simulink model "FieldControl_PID"  (R2021a)
settings: Solver=ode45  StartTime=0.0  StopTime=3  FixedStep=1e-5  MaxStep=1e-6  RelTol=1e-3
model workspace (MAT data in the model file):
  KI_s = 1
  KP_s = 1
undefined symbols (not defined in the file): DiscIntNeverNeededParam, Fsw, sigbuilder_block
libraries: simulink x2, spspowerguiLib x2
(part 1 of 2)
settings Model: SimulationMode=accelerator  OrderedModelArguments=off  Creator=AHMED  LastModifiedBy=AHMED
settings SolverCC: ZeroCrossAlgorithm=Adaptive
settings DebuggingCC: MaskedZcDiagnostic=none  IgnoredZcDiagnostic=none

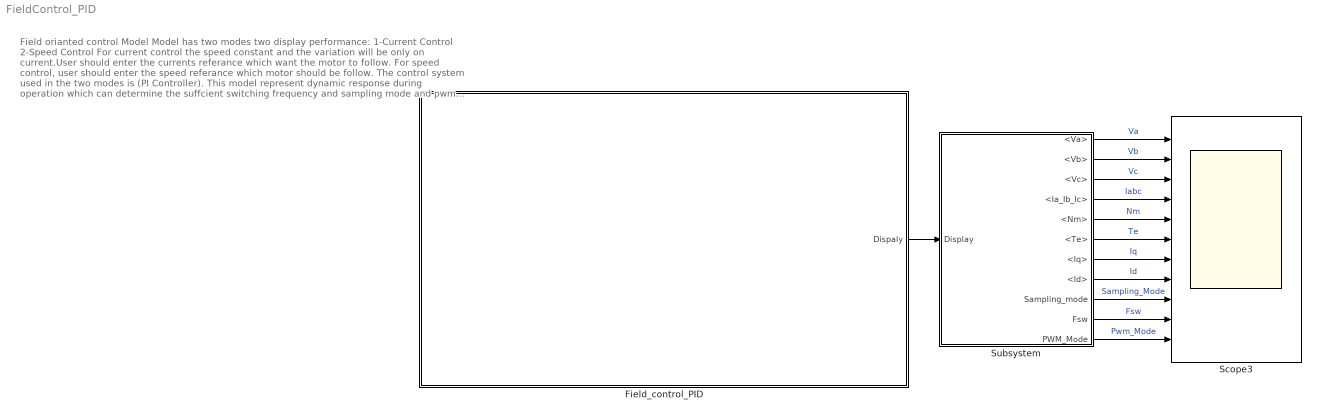
== system FieldControl_PID ==
  note: Field orianted control Model
      | Model has two modes two display performance:
      | 1-Current Control
      | 2-Speed Control
      | For current control the speed constant and the variation will be only on current.User should enter the currents referance which want the motor to follow.
      |
      | For speed control, user should enter the speed referance which motor should be follow.
      |
      | The control system used in the two modes is (PI Controller).
      |
      | This model represent dynamic response during operation which can determine the suffcient switching frequency and sampling mode and pwm generation technique.
      |
      | The dynamical behaviour according to the best performance and lower losses could be achieved.
      |
      | PWM generating techniques
      | 1-Space Vector Modulation(SVM)
      | 2-General Discontinous PWM (GDPWM)
      |
      | Sampling Modes
      | 1-Symmetrical Sampling Mode
      | 2-Asymmetrical Sampling Mode
      |
      | Selected switching frequency according fundmental frequency measured from the operating speed and it has low and high limits.
  Field_control_PID : Subsystem  Variant=on  mask{Mode=Speed_Control, Vdc=400, PWM_Mode=Auto, Sw2fund_Ration=50, Lower_Limit=4e3, Higher_Limit=10e3, Typee=Equations, TL=0.75, Nm_CC=1200}
      mask prompts: Mode "Control_System"; Vdc "DC voltage"; PWM_Mode "PWM_Generation_Mode"; Sw2fund_Ration "Switching to fund_ freq Ratio"; Lower_Limit "Lower Limit"; Typee "MTPA_System"; TL "Load Torque"; Nm_CC "Constant_Speed_RPM"
      mask TypeOptions Mode: Current_Control | Speed_Control
      mask TypeOptions PWM_Mode: SVM | DPWM | Auto
      mask TypeOptions Typee: Equations | Tables
      mask DialogControl DescGroupVar Prompt: FOC_PMSM_parameters
      mask DialogControl DescTextVar Prompt: Field orianted control with two modes of operation (current, speed)control. Each one has parametrs must be input before run
      mask DialogControl ParameterGroupVar Prompt: Control Type & Motor parameters
      mask DialogControl ParameterGroupVar2 Prompt: Frequency and sampling
      mask DialogControl ParameterGroupVar3 Prompt: Speed control parameters
      mask DialogControl ParameterGroupVar4 Prompt: Current control parameters
      mask Display: image('$imagefile'); % Use "Edit Image" on toolstrip to change.
  Scope3 : Scope  NumInputPorts=11
  Subsystem : Subsystem
      mask Display: image('$imagefile'); % Use "Edit Image" on toolstrip to change.
  wires:
  Field_control_PID/1(Dispaly) -> Subsystem/1(Display)
  Subsystem/1(<Va>) -> Scope3/1  "Va"
  Subsystem/2(<Vb>) -> Scope3/2  "Vb"
  Subsystem/3(<Vc>) -> Scope3/3  "Vc"
  Subsystem/4(<Ia_Ib_Ic>) -> Scope3/4  "Iabc"
  Subsystem/5(<Nm>) -> Scope3/5  "Nm"
  Subsystem/6(<Te>) -> Scope3/6  "Te"
  Subsystem/7(<Iq>) -> Scope3/7  "Iq"
  Subsystem/8(<Id>) -> Scope3/8  "Id"
  Subsystem/9(Sampling_mode) -> Scope3/9  "Sampling_Mode"
  Subsystem/10(Fsw) -> Scope3/10  "Fsw"
  Subsystem/11(PWM_Mode) -> Scope3/11  "Pwm_Mode"

== system FieldControl_PID/Field_control_PID ==
  Current_control : Subsystem  VariantControl=Mode==1
  Speed_control : Subsystem  VariantControl=Mode==2
  Dispaly : Outport

== system FieldControl_PID/Subsystem ==
  Display : Inport
  Bus Selector : BusSelector  OutputSignals=Va,Vb,Vc,Ia_Ib_Ic,Nm,Te,Iq,Id,sampling_Mode,Fswitching,PWM_Gen_Mode
  Constant : Constant  Value=2
  Constant1 : Constant
  Constant2 : Constant  Value=4e3
  Constant3 : Constant  Value=10e3
  Constant4 : Constant  Value=0
  Constant5 : Constant
  Mux : Mux  Inputs=3
  Mux1 : Mux  Inputs=3
  Mux2 : Mux  Inputs=3
  <Va> : Outport
  <Vb> : Outport  Port=2
  <Vc> : Outport  Port=3
  <Ia_Ib_Ic> : Outport  Port=4
  <Nm> : Outport  Port=5
  <Te> : Outport  Port=6
  <Iq> : Outport  Port=7
  <Id> : Outport  Port=8
  Sampling_mode : Outport  Port=9
  Fsw : Outport  Port=10
  PWM_Mode : Outport  Port=11
  wires:
  Bus Selector/10 -> Mux1/1  "<Fswitching>"
  Constant5/1 -> Mux2/3  "GDPWM"
  Constant2/1 -> Mux1/2  "Lower_Limit"
  Constant/1 -> Mux/2  "Symmetrical"
  Bus Selector/11 -> Mux2/1  "<PWM_Gen_Mode>"
  Constant1/1 -> Mux/3  "Asymmetrical"
  Bus Selector/6 -> <Te>/1  "<Te>"
  Constant3/1 -> Mux1/3  "Upper_Limit"
  Display/1 -> Bus Selector/1
  Bus Selector/9 -> Mux/1  "<sampling_Mode>"
  Constant4/1 -> Mux2/2  "SVM"
  Bus Selector/8 -> <Id>/1  "<Id>"
  Bus Selector/5 -> <Nm>/1  "<Nm>"
  Bus Selector/1 -> <Va>/1  "<Va>"
  Mux/1 -> Sampling_mode/1  "Sampling_mode"
  Bus Selector/3 -> <Vc>/1  "<Vc>"
  Bus Selector/4 -> <Ia_Ib_Ic>/1  "<Ia_Ib_Ic>"
  Bus Selector/2 -> <Vb>/1  "<Vb>"
  Bus Selector/7 -> <Iq>/1  "<Iq>"
  Mux1/1 -> Fsw/1
  Mux2/1 -> PWM_Mode/1  "PWM_Mode"

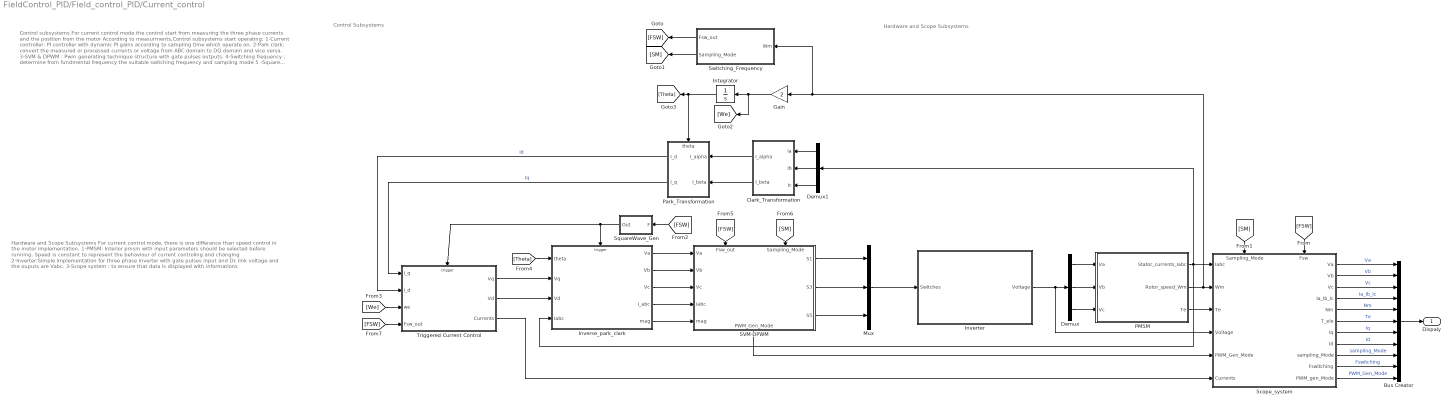
== system FieldControl_PID/Field_control_PID/Current_control ==
  note: Control subsystems
      | For current control mode the control start from measuring the three phase currents and the position from the motor
      | According to measurments,Control subsystems start operating:
      | 1-Current controller: PI controller with dynamic PI gains according to sampling time which operate on.
      |
      | 2-Park clark: convert the measured or processed currents or voltage
      | from ABC domain to DQ domain and vice versa.
      |
      | 3-SVM & DPWM : Pwm generating technique structure with gate pulses outputs.
      |
      | 4-Switching frequency : determine from fundmental frequency the suitable switching frequency and sampling mode
      |
      | 5 -Square Wave generator: with frequency input
  note: Hardware and Scope Subsystems
  note: Control Subsystems
  note: Hardware and Scope Subsystems
      | For current control mode, there is one differance than speed control in the motor implementation.
      | 1-PMSM: Interior pmsm with input parameters should be selected before running.
      | Speed is constant to represent the behaviour of current controling and changing
      |
      | 2-Inverter:Simple implementation for three phase inverter with gate pulses input and Dc link voltage and the ouputs are Vabc.
      |
      | 3-Scope system : to ensure that data is displayed with informations
  Bus Creator : BusCreator  Inputs=11
  Clark_Transformation : Subsystem
  Demux : Demux  Outputs=3
  Demux1 : Demux  Outputs=3
  Gain : Gain  Gain=2
  Integrator : Integrator
  Inverse_park_clark : Subsystem
  "Inverter " : Subsystem
      mask Display: image('E:\matlab_modules\FOC_PMSM\Final_1_FOC_PMSM\Images\WhatsApp Image 2024-10-21 at 22.54.49_e8a4c1c9.jpg'); % Use "Edit Image" on toolstrip to change.
  Mux : Mux  Inputs=3
  PMSM : Subsystem  mask{Ld=0.0057, Lq=0.0125, lamda_pm=0.123, R=1.2, P=4, J=0.0001, b=0}
      mask Display: image('$imagefile'); % Use "Edit Image" on toolstrip to change.
  Park_Transformation : Subsystem
      settings: PortSchema="{\"entries\":[{\"content\":{\"sides\":[{\"content\":{\"connectorIds\":[\"In1\",\"In2\"]},\"type\":\"ConnectorPlacement.EquallySpacedRectSide\",\"uuid\":\"a5303260-9056-4ba9-bf21-9d9e68c76aad\"},{\"content\":{\"connectorIds\":[\"Out1\",\"Out2\"],\"side\":\"RIGHT\"},\"type\":\"ConnectorPlacement.EquallySpacedRectSide\",\"uuid\":\"bf8eba39-f781-4672-b99d-9d1cb4b6396f\"},{\"content\":{\"connectorIds\":[\"In3\"],\"side\":\"TOP\"},\"type\":\"ConnectorPlacement.EquallySpacedRectSide\",\"uuid\":\"4985423e-053d-4914-82fe-b9dd9f427f0d\"},{\"content\":{\"connectorIds\":[],\"side\":\"BOTTOM\"},\"type\":\"ConnectorPlacement.EquallySpacedRectSide\",\"uuid\":\"0752c2be-c5bb-44b3-a6b0-4f5b66c2ccb1\"}]},\"type\":\"ConnectorPlacement.EquallySpacedConnector\",\"uuid\":\"0aeb7acd-9c9e-4bf3-9d65-4f157eb3bd0a\"}],\"packageUris\":[\"http://schema.mathworks.com/mf0/Connector/R2020b\"],\"version\":\"1.0\"}"
  SVM-DPWM : Subsystem
      settings: PortSchema="{\"entries\":[{\"content\":{\"sides\":[{\"content\":{\"connectorIds\":[\"In1\",\"In2\",\"In3\",\"In4\",\"In5\"]},\"type\":\"ConnectorPlacement.EquallySpacedRectSide\",\"uuid\":\"46ad86bc-2290-42eb-9805-a724d3d45e27\"},{\"content\":{\"connectorIds\":[\"Out1\",\"Out2\",\"Out3\"],\"side\":\"RIGHT\"},\"type\":\"ConnectorPlacement.EquallySpacedRectSide\",\"uuid\":\"f1ee6116-553b-4cc4-988e-efe9f7b6e0cc\"},{\"content\":{\"connectorIds\":[\"In6\",\"In7\"],\"side\":\"TOP\"},\"type\":\"ConnectorPlacement.EquallySpacedRectSide\",\"uuid\":\"0619aa55-dbb7-4591-ac57-1e3d225085e5\"},{\"content\":{\"connectorIds\":[\"Out4\"],\"side\":\"BOTTOM\"},\"type\":\"ConnectorPlacement.EquallySpacedRectSide\",\"uuid\":\"7325c7f4-f74c-41be-974a-a0e5e3a4c9b0\"}]},\"type\":\"ConnectorPlacement.EquallySpacedConnector\",\"uuid\":\"4aef647a-1044-4613-b672-2a7f7848e9d8\"}],\"packageUris\":[\"http://schema.mathworks.com/mf0/Connector/R2020b\"],\"version\":\"1.0\"}"
      mask Display: image('E:\matlab_modules\FOC_PMSM\Final_1_FOC_PMSM\Images\photo_2024-12-25_16-03-35.jpg'); % Use "Edit Image" on toolstrip to change.
  Scope_system : Subsystem
      settings: PortSchema="{\"entries\":[{\"content\":{\"sides\":[{\"content\":{\"connectorIds\":[\"In1\",\"In2\",\"In3\",\"In4\",\"In5\",\"In6\"]},\"type\":\"ConnectorPlacement.EquallySpacedRectSide\",\"uuid\":\"f5ff00d6-72d0-455a-b8b4-a2b5e0f936c9\"},{\"content\":{\"connectorIds\":[\"Out1\",\"Out2\",\"Out3\",\"Out4\",\"Out5\",\"Out6\",\"Out7\",\"Out8\",\"Out9\",\"Out10\",\"Out11\"],\"side\":\"RIGHT\"},\"type\":\"ConnectorPlacement.EquallySpacedRectSide\",\"uuid\":\"90221681-7e43-47d8-9ea8-4435eb27af9a\"},{\"content\":{\"connectorIds\":[\"In7\",\"In8\"],\"side\":\"TOP\"},\"type\":\"ConnectorPlacement.EquallySpacedRectSide\",\"uuid\":\"62fb04f8-341d-442a-bb15-2a5c062453bf\"}]},\"type\":\"ConnectorPlacement.EquallySpacedConnector\",\"uuid\":\"244d1d3d-d937-49d8-9876-c8777bd7e7cc\"}],\"packageUris\":[\"http://schema.mathworks.com/mf0/Connector/R2020b\"],\"version\":\"1.0\"}"
      mask Display: image('$imagefile'); % Use "Edit Image" on toolstrip to change.
  SquareWave_Gen : Subsystem
  Switching_Frequency : Subsystem
  Triggered Current Control : Subsystem  TreatAsAtomicUnit=on
  Dispaly : Outport
  wires:
  Demux1/3 -> Clark_Transformation/3(Ic)
  Demux1/1 -> Clark_Transformation/1(Ia)
  Scope_system/8("Id ") -> Bus Creator/8  "Id"
  Scope_system/7(Iq) -> Bus Creator/7  "Iq"
  Clark_Transformation/1(I_alpha) -> Park_Transformation/1(I_alpha)
  Scope_system/3(Vc) -> Bus Creator/3  "Vc"
  Clark_Transformation/2(I_beta) -> Park_Transformation/2(I_beta)
  Demux1/2 -> Clark_Transformation/2(Ib)
  Bus Creator/1 -> Dispaly/1
  Scope_system/1(Va) -> Bus Creator/1  "Va"
  Scope_system/4(Ia_Ib_Ic) -> Bus Creator/4  "Ia_Ib_Ic"
  Scope_system/2(Vb) -> Bus Creator/2  "Vb"
  Scope_system/5(Nm) -> Bus Creator/5  "Nm"
  Scope_system/6(T_ele) -> Bus Creator/6  "Te"
  Scope_system/9(sampling_Mode) -> Bus Creator/9  "sampling_Mode"
  Scope_system/10(Fswitching) -> Bus Creator/10  "Fswitching"
  Scope_system/11(PWM_gen_Mode) -> Bus Creator/11  "PWM_Gen_Mode"
  SVM-DPWM/1(S1) -> Mux/1
  SVM-DPWM/2(S3) -> Mux/2
  SVM-DPWM/3(S5) -> Mux/3
  Mux/1 -> "Inverter "/1("Switches ")
  "Inverter "/1("Voltage ") -> Scope_system/4("Voltage "), Demux/1
  Demux/1 -> PMSM/1(Va)
  Demux/2 -> PMSM/2(Vb)
  Demux/3 -> PMSM/3(Vc)
  Inverse_park_clark/1(Va) -> SVM-DPWM/1(Va)
  Inverse_park_clark/2(Vb) -> SVM-DPWM/2(Vb)
  Inverse_park_clark/3(Vc) -> SVM-DPWM/3(Vc)
  Inverse_park_clark/4(I_abc) -> SVM-DPWM/4(Iabc)
  Inverse_park_clark/5(mag) -> SVM-DPWM/5(mag)
  Triggered Current Control/1(Vq) -> Inverse_park_clark/2(Vq)
  Triggered Current Control/2(Vd) -> Inverse_park_clark/3(Vd)
  Gain/1 -> [We], Integrator/1
  Integrator/1 -> [Theta], Park_Transformation/3(theta)
  Switching_Frequency/1(Fsw_out) -> [FSW]
  Switching_Frequency/2(Sampling_Mode) -> [SM]
  [Theta] -> Inverse_park_clark/1(theta)
  Park_Transformation/2(I_q) -> Triggered Current Control/1(I_q)  "Iq"
  Park_Transformation/1(I_d) -> Triggered Current Control/2(I_d)  "Id"
  [FSW] -> SquareWave_Gen/1(F)
  SquareWave_Gen/1(Out) -> Inverse_park_clark/Trigger, Triggered Current Control/Trigger
  [We] -> Triggered Current Control/3(we)
  [SM] -> Scope_system/7(Sampling_Mode)
  [FSW] -> Scope_system/8(Fsw)
  [SM] -> SVM-DPWM/7(Sampling_Mode)
  [FSW] -> SVM-DPWM/6(Fsw_out)
  [FSW] -> Triggered Current Control/4(Fsw_out)
  PMSM/1(Stator_currents_Iabc) -> Inverse_park_clark/4(Iabc), Scope_system/1(Iabc), Demux1/1
  PMSM/2(Rotor_speed_Wm) -> Switching_Frequency/1(Wm), Gain/1, Scope_system/2(Wm)
  PMSM/3(Te) -> Scope_system/3(Te)
  Triggered Current Control/3(Currents) -> Scope_system/6(Currents)
  SVM-DPWM/4(PWM_Gen_Mode) -> Scope_system/5(PWM_Gen_Mode)

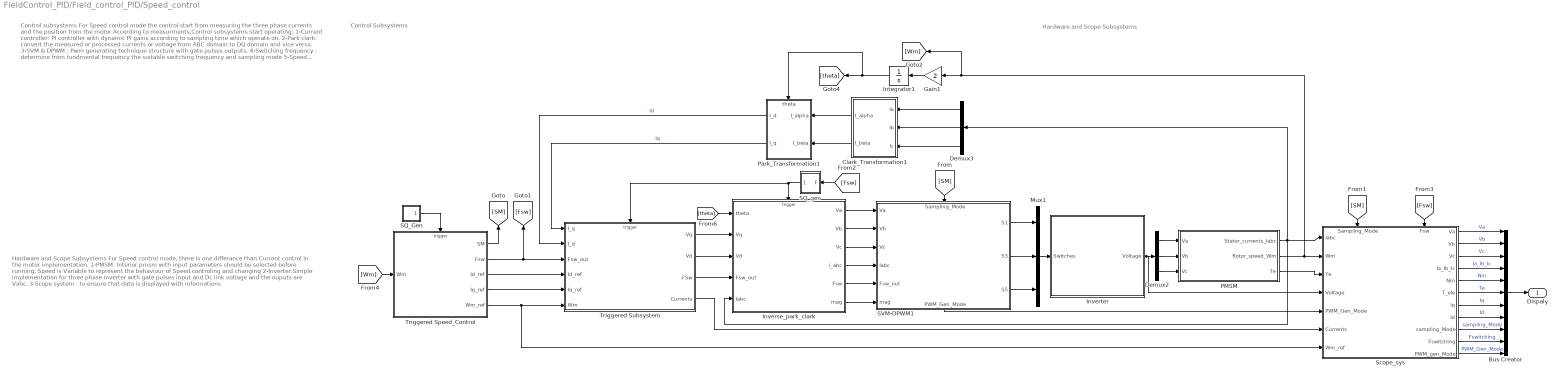
== system FieldControl_PID/Field_control_PID/Speed_control ==
  note: Hardware and Scope Subsystems
  note: Control Subsystems
  note: Control subsystems
      | For Speed control mode the control start from measuring the three phase currents and the position from the motor
      | According to measurments,Control subsystems start operating:
      | 1-Current controller: PI controller with dynamic PI gains according to sampling time which operate on.
      |
      | 2-Park clark: convert the measured or processed currents or voltage
      | from ABC domain to DQ domain and vice versa.
      |
      | 3-SVM & DPWM : Pwm generating technique structure with gate pulses outputs.
      |
      | 4-Switching frequency : determine from fundmental frequency the suitable switching frequency and sampling mode
      |
      | 5-Speed Controller: PI controller with constant PI gains.
      |
      | 6-Square Wave generator: with frequency input
  note: Hardware and Scope Subsystems
      | For Speed control mode, there is one differance than Current control in the motor implementation.
      | 1-PMSM: Interior pmsm with input parameters should be selected before running.
      | Speed is Variable to represent the behaviour of Speed controling and changing
      |
      | 2-Inverter:Simple implementation for three phase inverter with gate pulses input and Dc link voltage and the ouputs are Vabc.
      |
      | 3-Scope system : to ensure that data is displayed with informations
  Bus Creator : BusCreator  Inputs=11
  Clark_Transformation1 : Subsystem
  Demux2 : Demux  Outputs=3
  Demux3 : Demux  Outputs=3
  Gain1 : Gain  Gain=2
  Integrator1 : Integrator
  Inverse_park_clark : Subsystem
  "Inverter " : Subsystem
      mask Display: image('$imagefile'); % Use "Edit Image" on toolstrip to change.
  Mux1 : Mux  Inputs=3
  PMSM : Subsystem  mask{Ld=0.0057, Lq=0.0125, lamda_pm=0.123, R=1.2, P=4, J=0.0001, b=0}
      mask Display: image('$imagefile'); % Use "Edit Image" on toolstrip to change.
  Park_Transformation1 : Subsystem
      settings: PortSchema="{\"entries\":[{\"content\":{\"sides\":[{\"content\":{\"connectorIds\":[\"In1\",\"In2\"]},\"type\":\"ConnectorPlacement.EquallySpacedRectSide\",\"uuid\":\"a5303260-9056-4ba9-bf21-9d9e68c76aad\"},{\"content\":{\"connectorIds\":[\"Out1\",\"Out2\"],\"side\":\"RIGHT\"},\"type\":\"ConnectorPlacement.EquallySpacedRectSide\",\"uuid\":\"bf8eba39-f781-4672-b99d-9d1cb4b6396f\"},{\"content\":{\"connectorIds\":[\"In3\"],\"side\":\"TOP\"},\"type\":\"ConnectorPlacement.EquallySpacedRectSide\",\"uuid\":\"4985423e-053d-4914-82fe-b9dd9f427f0d\"},{\"content\":{\"connectorIds\":[],\"side\":\"BOTTOM\"},\"type\":\"ConnectorPlacement.EquallySpacedRectSide\",\"uuid\":\"0752c2be-c5bb-44b3-a6b0-4f5b66c2ccb1\"}]},\"type\":\"ConnectorPlacement.EquallySpacedConnector\",\"uuid\":\"0aeb7acd-9c9e-4bf3-9d65-4f157eb3bd0a\"}],\"packageUris\":[\"http://schema.mathworks.com/mf0/Connector/R2020b\"],\"version\":\"1.0\"}"
  SQ_Gen : Subsystem
  SQ_gen : Subsystem
  SVM-DPWM1 : Subsystem
      settings: PortSchema="{\"entries\":[{\"content\":{\"sides\":[{\"content\":{\"connectorIds\":[\"In1\",\"In2\",\"In3\",\"In4\",\"In5\",\"In6\"]},\"type\":\"ConnectorPlacement.EquallySpacedRectSide\",\"uuid\":\"46ad86bc-2290-42eb-9805-a724d3d45e27\"},{\"content\":{\"connectorIds\":[\"Out1\",\"Out2\",\"Out3\"],\"side\":\"RIGHT\"},\"type\":\"ConnectorPlacement.EquallySpacedRectSide\",\"uuid\":\"f1ee6116-553b-4cc4-988e-efe9f7b6e0cc\"},{\"content\":{\"connectorIds\":[\"In7\"],\"side\":\"TOP\"},\"type\":\"ConnectorPlacement.EquallySpacedRectSide\",\"uuid\":\"0619aa55-dbb7-4591-ac57-1e3d225085e5\"},{\"content\":{\"connectorIds\":[\"Out4\"],\"side\":\"BOTTOM\"},\"type\":\"ConnectorPlacement.EquallySpacedRectSide\",\"uuid\":\"7325c7f4-f74c-41be-974a-a0e5e3a4c9b0\"}]},\"type\":\"ConnectorPlacement.EquallySpacedConnector\",\"uuid\":\"4aef647a-1044-4613-b672-2a7f7848e9d8\"}],\"packageUris\":[\"http://schema.mathworks.com/mf0/Connector/R2020b\"],\"version\":\"1.0\"}"
      mask Display: image('$imagefile'); % Use "Edit Image" on toolstrip to change.
  Scope_sys : Subsystem
      settings: PortSchema="{\"entries\":[{\"content\":{\"sides\":[{\"content\":{\"connectorIds\":[\"In1\",\"In2\",\"In3\",\"In4\",\"In5\",\"In6\",\"In7\"]},\"type\":\"ConnectorPlacement.EquallySpacedRectSide\",\"uuid\":\"f5ff00d6-72d0-455a-b8b4-a2b5e0f936c9\"},{\"content\":{\"connectorIds\":[\"Out1\",\"Out2\",\"Out3\",\"Out4\",\"Out5\",\"Out6\",\"Out7\",\"Out8\",\"Out9\",\"Out10\",\"Out11\"],\"side\":\"RIGHT\"},\"type\":\"ConnectorPlacement.EquallySpacedRectSide\",\"uuid\":\"90221681-7e43-47d8-9ea8-4435eb27af9a\"},{\"content\":{\"connectorIds\":[\"In8\",\"In9\"],\"side\":\"TOP\"},\"type\":\"ConnectorPlacement.EquallySpacedRectSide\",\"uuid\":\"62fb04f8-341d-442a-bb15-2a5c062453bf\"}]},\"type\":\"ConnectorPlacement.EquallySpacedConnector\",\"uuid\":\"244d1d3d-d937-49d8-9876-c8777bd7e7cc\"}],\"packageUris\":[\"http://schema.mathworks.com/mf0/Connector/R2020b\"],\"version\":\"1.0\"}"
      mask Display: image('$imagefile'); % Use "Edit Image" on toolstrip to change.
  Triggered Speed_Control : Subsystem  TreatAsAtomicUnit=on
  Triggered Subsystem : Subsystem  TreatAsAtomicUnit=on
  Dispaly : Outport
  wires:
  "Inverter "/1("Voltage ") -> Scope_sys/4("Voltage "), Demux2/1
  Demux3/1 -> Clark_Transformation1/1(Ia)
  Scope_sys/8("Id ") -> Bus Creator/8  "Id"
  Scope_sys/7(Iq) -> Bus Creator/7  "Iq"
  Demux3/3 -> Clark_Transformation1/3(Ic)
  Scope_sys/6(T_ele) -> Bus Creator/6  "Te"
  Scope_sys/3(Vc) -> Bus Creator/3  "Vc"
  Scope_sys/5(Nm) -> Bus Creator/5  "Nm"
  Scope_sys/2(Vb) -> Bus Creator/2  "Vb"
  Scope_sys/10(Fswitching) -> Bus Creator/10  "Fswitching"
  Scope_sys/1(Va) -> Bus Creator/1  "Va"
  Mux1/1 -> "Inverter "/1("Switches ")
  Demux3/2 -> Clark_Transformation1/2(Ib)
  Clark_Transformation1/1(I_alpha) -> Park_Transformation1/1(I_alpha)
  Scope_sys/9(sampling_Mode) -> Bus Creator/9  "sampling_Mode"
  Clark_Transformation1/2(I_beta) -> Park_Transformation1/2(I_beta)
  Bus Creator/1 -> Dispaly/1
  Scope_sys/4(Ia_Ib_Ic) -> Bus Creator/4  "Ia_Ib_Ic"
  [SM] -> SVM-DPWM1/7(Sampling_Mode)
  [SM] -> Scope_sys/8(Sampling_Mode)
  SQ_gen/1(Cs) -> Triggered Subsystem/Trigger, Inverse_park_clark/Trigger
  [Fsw] -> SQ_gen/1(F)
  [Fsw] -> Scope_sys/9(Fsw)
  [theta] -> Inverse_park_clark/1(theta)
  Scope_sys/11(PWM_gen_Mode) -> Bus Creator/11  "PWM_Gen_Mode"
  PMSM/1(Stator_currents_Iabc) -> Demux3/1, Scope_sys/1(Iabc), Inverse_park_clark/5(Iabc)
  PMSM/2(Rotor_speed_Wm) -> [Wm], Gain1/1, Scope_sys/2(Wm)
  PMSM/3(Te) -> Scope_sys/3(Te)
  Demux2/1 -> PMSM/1(Va)
  Demux2/2 -> PMSM/2(Vb)
  Demux2/3 -> PMSM/3(Vc)
  SVM-DPWM1/1(S1) -> Mux1/1
  SVM-DPWM1/2(S3) -> Mux1/2
  SVM-DPWM1/3(S5) -> Mux1/3
  Inverse_park_clark/1(Va) -> SVM-DPWM1/1(Va)
  Inverse_park_clark/2(Vb) -> SVM-DPWM1/2(Vb)
  Inverse_park_clark/3(Vc) -> SVM-DPWM1/3(Vc)
  Inverse_park_clark/4(i_abc) -> SVM-DPWM1/4(Iabc)
  Inverse_park_clark/5(Fsw) -> SVM-DPWM1/5(Fsw_out)
  Inverse_park_clark/6(mag) -> SVM-DPWM1/6(mag)
  Triggered Subsystem/1(Vq) -> Inverse_park_clark/2(Vq)
  Triggered Subsystem/2(Vd) -> Inverse_park_clark/3(Vd)
  Triggered Subsystem/3(FSw) -> Inverse_park_clark/4(Fsw_out)
  Integrator1/1 -> Park_Transformation1/3(theta), [theta]
  Gain1/1 -> Integrator1/1
  Triggered Subsystem/4(Currents) -> Scope_sys/6(Currents)
  SVM-DPWM1/4(PWM_Gen_Mode) -> Scope_sys/5(PWM_Gen_Mode)
  Triggered Speed_Control/2(Fsw) -> [Fsw], Triggered Subsystem/3(Fsw_out)
  Triggered Speed_Control/3(Id_ref) -> Triggered Subsystem/4(Id_ref)
  Triggered Speed_Control/4(Iq_ref) -> Triggered Subsystem/5(Iq_ref)
  Triggered Speed_Control/5(Wm_ref) -> Triggered Subsystem/6(Wm), Scope_sys/7(Wm_ref)
  Triggered Speed_Control/1(SM) -> [SM]
  [Wm] -> Triggered Speed_Control/1(Wm)
  Park_Transformation1/2(I_q) -> Triggered Subsystem/1(I_q)  "Iq"
  Park_Transformation1/1(I_d) -> Triggered Subsystem/2(I_d)  "Id"
  SQ_Gen/1(Cs) -> Triggered Speed_Control/Trigger

== system FieldControl_PID/Field_control_PID/Current_control/Clark_Transformation ==
  Ia : Inport
  Ib : Inport  Port=2
  Ic : Inport  Port=3
  Add : Sum  Inputs=+++
  Add1 : Sum
  Gain : Gain  Gain=-0.5
  Gain1 : Gain  Gain=-0.5
  Gain2 : Gain  Gain=2/3
  Gain3 : Gain  Gain=sqrt(3)/2
  Gain4 : Gain  Gain=-sqrt(3)/2
  Gain5 : Gain  Gain=2/3
  I_alpha : Outport
  I_beta : Outport  Port=2
  wires:
  Gain5/1 -> I_beta/1
  Add1/1 -> Gain5/1
  Gain3/1 -> Add1/1
  Gain4/1 -> Add1/2
  Gain2/1 -> I_alpha/1
  Add/1 -> Gain2/1
  Ia/1 -> Add/1
  Gain1/1 -> Add/3
  Gain/1 -> Add/2
  Ic/1 -> Gain1/1, Gain4/1
  Ib/1 -> Gain/1, Gain3/1

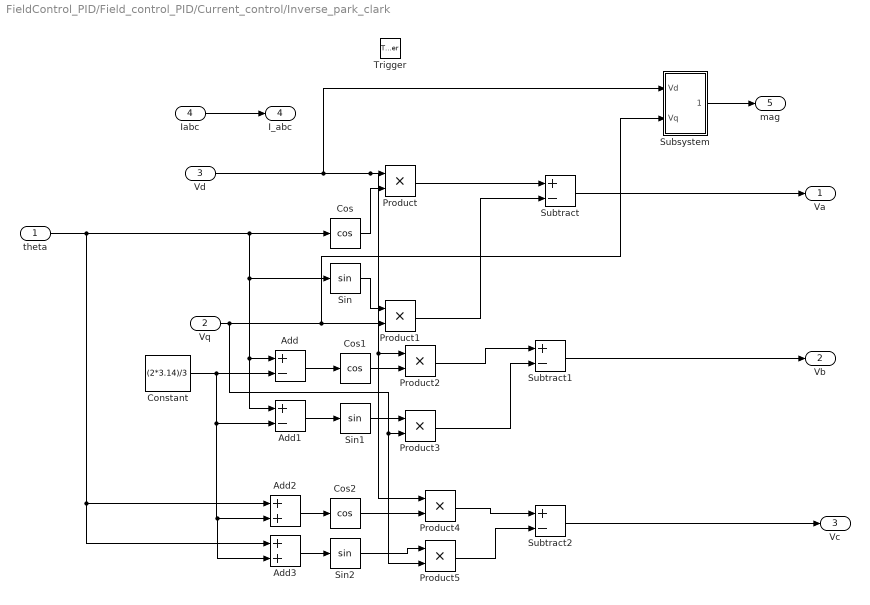
== system FieldControl_PID/Field_control_PID/Current_control/Inverse_park_clark ==
  theta : Inport
  Vq : Inport  Port=2
  Vd : Inport  Port=3
  Iabc : Inport  Port=4
  Trigger : TriggerPort  VariantControl=(inherit)
  Add : Sum  Inputs=+-
  Add1 : Sum  Inputs=+-
  Add2 : Sum
  Add3 : Sum
  Constant : Constant  Value=(2*3.14)/3
  Cos : Trigonometry  Operator=cos
  Cos1 : Trigonometry  Operator=cos
  Cos2 : Trigonometry  Operator=cos
  Product{,1..5} (6 alike) : Product
  Sin : Trigonometry
  Sin1 : Trigonometry
  Sin2 : Trigonometry
  Subsystem : Subsystem
  Subtract : Sum  Inputs=+-
  Subtract1 : Sum  Inputs=+-
  Subtract2 : Sum  Inputs=+-
  Va : Outport
  Vb : Outport  Port=2
  Vc : Outport  Port=3
  I_abc : Outport  Port=4
  mag : Outport  Port=5
  wires:
  Add3/1 -> Sin2/1
  Add2/1 -> Cos2/1
  Sin2/1 -> Product5/1
  Cos2/1 -> Product4/2
  Product5/1 -> Subtract2/2
  Product4/1 -> Subtract2/1
  Subtract2/1 -> Vc/1
  Constant/1 -> Add/2, Add1/2, Add2/2, Add3/2
  Subtract1/1 -> Vb/1
  Product3/1 -> Subtract1/2
  Product2/1 -> Subtract1/1
  Sin1/1 -> Product3/1
  Cos1/1 -> Product2/2
  Add1/1 -> Sin1/1
  Add/1 -> Cos1/1
  Product1/1 -> Subtract/2
  Sin/1 -> Product1/1
  Vq/1 -> Subsystem/2(Vq), Product1/2, Product3/2, Product5/2
  Product/1 -> Subtract/1
  Cos/1 -> Product/2
  Vd/1 -> Subsystem/1(Vd), Product/1, Product2/1, Product4/1
  theta/1 -> Sin/1, Add/1, Add1/1, Cos/1, Add2/1, Add3/1
  Subtract/1 -> Va/1
  Iabc/1 -> I_abc/1
  Subsystem/1(mag) -> mag/1

== system FieldControl_PID/Field_control_PID/Current_control/Inverter  ==
  "Switches " : Inport
  Fcn : Fcn  Expr=Vdc/3*(2*u(1)-u(2)-u(3))
  Fcn1 : Fcn  Expr=Vdc/3*(2*u(2)-u(1)-u(3))
  Fcn2 : Fcn  Expr=Vdc/3*(2*u(3)-u(2)-u(1))
  Mux1 : Mux  Inputs=3
  "Voltage " : Outport  VectorParamsAs1DForOutWhenUnconnected=off
  wires:
  Fcn2/1 -> Mux1/3
  Fcn/1 -> Mux1/1
  "Switches "/1 -> Fcn/1, Fcn1/1, Fcn2/1
  Fcn1/1 -> Mux1/2
  Mux1/1 -> "Voltage "/1

== system FieldControl_PID/Field_control_PID/Current_control/PMSM ==
  Va : Inport
  Vb : Inport  Port=2
  Vc : Inport  Port=3
  Clark_Transformation : Subsystem
  Electrical_system1 : Subsystem
  Gain : Gain  Gain=P/2
  Gain1 : Gain  Gain=(2*pi)/60
  Integrator : Integrator
  Inverse_park_clark : Subsystem
  Mux : Mux  Inputs=3
  Nm : Constant  Value=Nm_CC
  Park_Transformation : Subsystem
      settings: PortSchema="{\"entries\":[{\"content\":{\"sides\":[{\"content\":{\"connectorIds\":[\"In1\",\"In2\"]},\"type\":\"ConnectorPlacement.EquallySpacedRectSide\",\"uuid\":\"a5303260-9056-4ba9-bf21-9d9e68c76aad\"},{\"content\":{\"connectorIds\":[\"Out1\",\"Out2\"],\"side\":\"RIGHT\"},\"type\":\"ConnectorPlacement.EquallySpacedRectSide\",\"uuid\":\"bf8eba39-f781-4672-b99d-9d1cb4b6396f\"},{\"content\":{\"connectorIds\":[],\"side\":\"TOP\"},\"type\":\"ConnectorPlacement.EquallySpacedRectSide\",\"uuid\":\"4985423e-053d-4914-82fe-b9dd9f427f0d\"},{\"content\":{\"connectorIds\":[\"In3\"],\"side\":\"BOTTOM\"},\"type\":\"ConnectorPlacement.EquallySpacedRectSide\",\"uuid\":\"0752c2be-c5bb-44b3-a6b0-4f5b66c2ccb1\"}]},\"type\":\"ConnectorPlacement.EquallySpacedConnector\",\"uuid\":\"0aeb7acd-9c9e-4bf3-9d65-4f157eb3bd0a\"}],\"packageUris\":[\"http://schema.mathworks.com/mf0/Connector/R2020b\"],\"version\":\"1.0\"}"
  Scope : Scope  NumInputPorts=2
  Scope1 : Scope  NumInputPorts=2
  Torque_system : Subsystem
  Stator_currents_Iabc : Outport
  Rotor_speed_Wm : Outport  Port=2
  Te : Outport  Port=3
  wires:
  Gain1/1 -> Gain/1, Rotor_speed_Wm/1
  Nm/1 -> Gain1/1
  Mux/1 -> Stator_currents_Iabc/1
  Inverse_park_clark/3(Ic) -> Mux/3  "Ic"
  Inverse_park_clark/2(Ib) -> Mux/2  "Ib"
  Inverse_park_clark/1(Ia) -> Mux/1  "Ia"
  Integrator/1 -> Park_Transformation/3(theta), Inverse_park_clark/1(theta)  "Rotor_angle_theta_elec"
  Gain/1 -> Integrator/1, Electrical_system1/3(W_e)  "We"
  Torque_system/1(Te) -> Te/1  "Te"
  Electrical_system1/2(I_q) -> Torque_system/2(I_q), Inverse_park_clark/2(Iq), Scope/1  "Iq"
  Electrical_system1/1(I_d) -> Inverse_park_clark/3(Id), Scope/2, Torque_system/1(I_d)  "Id"
  Park_Transformation/2(V_q) -> Scope1/2, Electrical_system1/2(V_q)  "Vq"
  Park_Transformation/1(V_d) -> Scope1/1, Electrical_system1/1(V_d)  "Vd"
  Clark_Transformation/2(V_beta) -> Park_Transformation/2(V_beta)
  Clark_Transformation/1(V_alpha) -> Park_Transformation/1(V_alpha)
  Vc/1 -> Clark_Transformation/3(Vc)
  Vb/1 -> Clark_Transformation/2(Vb)
  Va/1 -> Clark_Transformation/1(Va)

== system FieldControl_PID/Field_control_PID/Current_control/Park_Transformation ==
  I_alpha : Inport
  I_beta : Inport  Port=2
  theta : Inport  Port=3
  Add : Sum
  Add1 : Sum
  Cos : Trigonometry  Operator=cos
  Cos1 : Trigonometry
  Gain : Gain  Gain=-1
  Product{,1..3} (4 alike) : Product
  I_d : Outport
  I_q : Outport  Port=2
  wires:
  Add1/1 -> I_q/1
  Product3/1 -> Add1/2
  Gain/1 -> Add1/1
  Product2/1 -> Gain/1
  Add/1 -> I_d/1
  Product1/1 -> Add/2
  Product/1 -> Add/1
  I_beta/1 -> Product1/2, Product3/1
  Cos1/1 -> Product1/1, Product2/2
  Cos/1 -> Product/2, Product3/2
  I_alpha/1 -> Product/1, Product2/1
  theta/1 -> Cos/1, Cos1/1

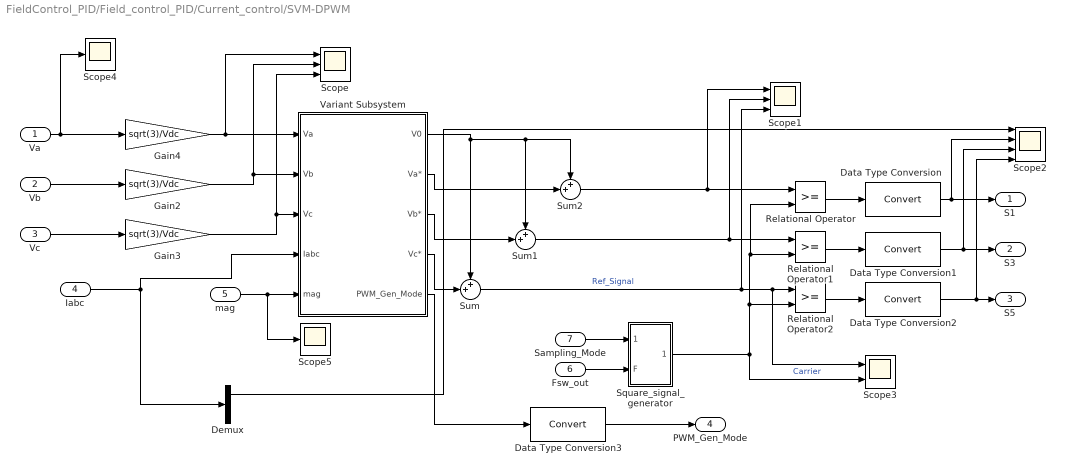
== system FieldControl_PID/Field_control_PID/Current_control/SVM-DPWM ==
  Va : Inport
  Vb : Inport  Port=2
  Vc : Inport  Port=3
  Iabc : Inport  Port=4
  mag : Inport  Port=5
  Fsw_out : Inport  Port=6
  Sampling_Mode : Inport  Port=7
  Data Type Conversion{,1..3} (4 alike) : DataTypeConversion
  Demux : Demux  Outputs=3
  Gain2 : Gain  Gain=sqrt(3)/Vdc
  Gain3 : Gain  Gain=sqrt(3)/Vdc
  Gain4 : Gain  Gain=sqrt(3)/Vdc
  Relational Operator : RelationalOperator  OutDataTypeStr=boolean  RndMeth=Simplest
  Relational Operator1 : RelationalOperator  OutDataTypeStr=boolean  RndMeth=Simplest
  Relational Operator2 : RelationalOperator  OutDataTypeStr=boolean  RndMeth=Simplest
  Scope : Scope  NumInputPorts=3
  Scope1 : Scope  NumInputPorts=3
  Scope2 : Scope  NumInputPorts=4
  Scope3 : Scope  NumInputPorts=2
  Scope4 : Scope
  Scope5 : Scope
  Square_signal_generator : Subsystem
  Sum : Sum  Inputs=++|
  Sum1 : Sum  Inputs=++|
  Sum2 : Sum  Inputs=++|
  Variant Subsystem : Subsystem  Variant=on
  S1 : Outport
  S3 : Outport  Port=2
  S5 : Outport  Port=3
  PWM_Gen_Mode : Outport  Port=4  OutDataTypeStr=double
  wires:
  Data Type Conversion/1 -> Scope2/2, S1/1
  Data Type Conversion1/1 -> Scope2/3, S3/1
  Data Type Conversion2/1 -> Scope2/4, S5/1
  Relational Operator/1 -> Data Type Conversion/1
  Relational Operator1/1 -> Data Type Conversion1/1
  Relational Operator2/1 -> Data Type Conversion2/1
  Sum/1 -> Scope1/3, Scope3/1, Relational Operator2/1  "Ref_Signal"
  Sum1/1 -> Relational Operator1/1, Scope1/2
  Sum2/1 -> Relational Operator/1, Scope1/1
  Square_signal_generator/1(Output) -> Relational Operator/2, Relational Operator1/2, Relational Operator2/2, Scope3/2  "Carrier"
  Variant Subsystem/1(V0) -> Sum2/1, Sum1/1, Sum/1
  Va/1 -> Scope4/1, Gain4/1
  Vb/1 -> Gain2/1
  Vc/1 -> Gain3/1
  Variant Subsystem/2(Va*) -> Sum2/2
  Variant Subsystem/3(Vb*) -> Sum1/2
  Variant Subsystem/4(Vc*) -> Sum/2
  Sampling_Mode/1 -> Square_signal_generator/1(Mode)
  Fsw_out/1 -> Square_signal_generator/2(F)
  Iabc/1 -> Variant Subsystem/4(Iabc), Demux/1
  Gain4/1 -> Scope/1, Variant Subsystem/1(Va)
  Gain2/1 -> Scope/2, Variant Subsystem/2(Vb)
  Gain3/1 -> Scope/3, Variant Subsystem/3(Vc)
  Demux/1 -> Scope2/1
  mag/1 -> Scope5/1, Variant Subsystem/5(mag)
  Variant Subsystem/5(PWM_Gen_Mode) -> Data Type Conversion3/1
  Data Type Conversion3/1 -> PWM_Gen_Mode/1

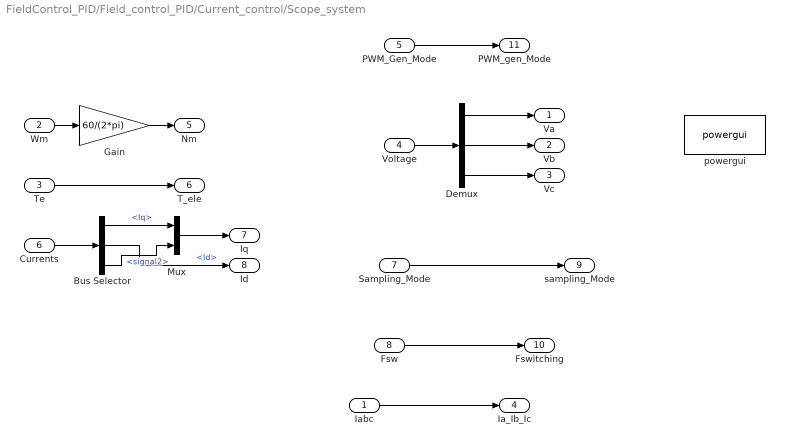
== system FieldControl_PID/Field_control_PID/Current_control/Scope_system ==
  Iabc : Inport
  Wm : Inport  Port=2
  Te : Inport  Port=3
  "Voltage " : Inport  Port=4
  PWM_Gen_Mode : Inport  Port=5
  Currents : Inport  Port=6
  Sampling_Mode : Inport  Port=7
  Fsw : Inport  Port=8
  Bus Selector : BusSelector  OutputSignals=Iq,Id,signal2
  Demux : Demux  Outputs=3
  Gain : Gain  Gain=60/(2*pi)
  Mux : Mux  Inputs=2
  powergui : spspowerguiLib/powergui  Priority=1  SimulationMode=Continuous  SampleTime=50e-6  frequency=60  Iterations=50  frequencyindice=60  Pbase=100e6  ErrMax=1e-4  UnitsV=kV  UnitsW=MW  buscounter=0  FunctionMessages=off  echomessages=off  EnableUseOfTLC=off  CurrentSourceSwitches=off  DisableSnubberDevices=off  DisableRonSwitches=off  DisableVfSwitches=off  DisplayEquations=off  AutomaticDiscreteSolvers=off  SolverType=Tustin/Backward Euler (TBE)  Interpol=off  ExternalGateDelay=off  methode=off  Ts=100  x0status=blocks  SPID=on  SwTol=0  HookPort=off  NonlinearTolerance=1e-4  nMaxIteration=100  ContinueOnMaxIteration=off  RestoreLinks=warning  ResistiveCurrentMeasurement=off  Frange=[0:2:500]  Ylog=off  Xlog=on  ShowGrid=off  save=off  variable=ZData  structure=0  ZoomFFT=off  StartTime=0.0  cycles=1  DisplayStyle=1  fundamental=60  FreqAxis=off  MaxFrequency=1000  frequencyindicesteady=1  RmsSteady=1  display=off
  Va : Outport
  Vb : Outport  Port=2
  Vc : Outport  Port=3
  Ia_Ib_Ic : Outport  Port=4
  Nm : Outport  Port=5
  T_ele : Outport  Port=6
  Iq : Outport  Port=7
  "Id " : Outport  Port=8
  sampling_Mode : Outport  Port=9
  Fswitching : Outport  Port=10
  PWM_gen_Mode : Outport  Port=11
  wires:
  Mux/1 -> Iq/1
  Bus Selector/2 -> "Id "/1  "<Id>"
  Bus Selector/3 -> Mux/2  "<signal2>"
  Bus Selector/1 -> Mux/1  "<Iq>"
  Currents/1 -> Bus Selector/1
  Te/1 -> T_ele/1
  Gain/1 -> Nm/1
  Wm/1 -> Gain/1
  Iabc/1 -> Ia_Ib_Ic/1
  Demux/3 -> Vc/1
  Demux/2 -> Vb/1
  Demux/1 -> Va/1
  "Voltage "/1 -> Demux/1
  Fsw/1 -> Fswitching/1
  Sampling_Mode/1 -> sampling_Mode/1
  PWM_Gen_Mode/1 -> PWM_gen_Mode/1

== system FieldControl_PID/Field_control_PID/Current_control/SquareWave_Gen ==
  F : Inport
  Clock : Clock
  Constant : Constant
  Divide : Product  Inputs=*/
  Gain1 : Gain  Gain=0.5
  Gain2 : Gain
  Mod : Math  Operator=mod  SaturateOnIntegerOverflow=on
  Relational Operator : RelationalOperator  Operator=<=  OutDataTypeStr=boolean  RndMeth=Simplest
  Out : Outport
  wires:
  Relational Operator/1 -> Out/1
  Gain1/1 -> Relational Operator/2
  Constant/1 -> Divide/1
  Clock/1 -> Mod/1
  Divide/1 -> Mod/2, Gain1/1
  Gain2/1 -> Divide/2
  F/1 -> Gain2/1
  Mod/1 -> Relational Operator/1

== system FieldControl_PID/Field_control_PID/Current_control/Switching_Frequency ==
  Wm : Inport
  Chart : Stateflow chart  TreatAsAtomicUnit=on
  Constant1 : Constant  Value=Lower_Limit
  Constant3 : Constant  Value=Higher_Limit
  Gain : Gain  Gain=Sw2fund_Ration
  N2F : Gain  Gain=4/120
  Wm2N : Gain  Gain=60/(2*pi)
  Fsw_out : Outport
  Sampling_Mode : Outport  Port=2
  wires:
  Wm2N/1 -> N2F/1
  Wm/1 -> Wm2N/1
  N2F/1 -> Gain/1
  Gain/1 -> Chart/3(Fsw_input)
  Chart/1(Fsw_out) -> Fsw_out/1
  Chart/2(Sampling_Mode) -> Sampling_Mode/1
  Constant3/1 -> Chart/2(High_Limit)
  Constant1/1 -> Chart/1(Low_limit)

== system FieldControl_PID/Field_control_PID/Current_control/Triggered Current Control ==
  I_q : Inport
  I_d : Inport  Port=2
  we : Inport  Port=3
  Fsw_out : Inport  Port=4
  Trigger : TriggerPort  VariantControl=(inherit)
  Bus Creator : BusCreator  Inputs=3
  FFW : Subsystem
  Gain : Gain
  Gain1 : Gain
  Gain2 : Gain
  I_d_ref : Constant  Value=0
  PID_2 : Subsystem
  PID_3 : Subsystem
  Saturation1 : Saturate  UpperLimit=Vdc/sqrt(3)  LowerLimit=-Vdc/sqrt(3)
  Saturation3 : Saturate  UpperLimit=Vdc/sqrt(3)  LowerLimit=-Vdc/sqrt(3)
  Signal Builder1 : Subsystem  Tag=STV Subsys  LoadFcn=sigbuilder_block('load');  StartFcn=sigbuilder_block('start');  StopFcn=sigbuilder_block('stop');  ClipboardFcn=sigbuilder_block('clipboard');  mask(Sigbuilder block){tuvar=[0:10]}
      mask help: Simulink:masks:SigbuilderBlock_MD
      mask init:
      | if ~strcmp(get_param(bdroot(gcbh),'SimulationStatus'),'stopped') tuvar = sigbuilder_block('maskInit'); end
      settings: CopyFcn=sigbuilder_block('copy');  DeleteFcn=sigbuilder_block('delete');  ModelCloseFcn=sigbuilder_block('modelClose');  PreSaveFcn=sigbuilder_block('preSave');  PauseFcn=sigbuilder_block('pause');  ContinueFcn=sigbuilder_block('continue');  NameChangeFcn=sigbuilder_block('namechange');  OpenFcn=sigbuilder_block('open',[5.4 30 1141.2 522.6 ]);  CloseFcn=sigbuilder_block('close');
      mask Display: plot(0, 0, 100, 100,[2, 2, 32, 32, 2], [68, 8, 8, 68, 68],[32, 2], [38, 38], [32, 19, 2],[53, 60, 44], [32, 17, 17, 2],[16, 16, 31, 31]);txt = getActiveGroup(gcbh);text(2, 100, txt,'verticalAlignment', 'top');
  Sum1 : Sum  Inputs=-+|
  Sum2 : Sum  Inputs=|+-
  Sum3 : Sum  Inputs=|++
  Sum4 : Sum  Inputs=-+|
  Vq : Outport
  Vd : Outport  Port=2
  Currents : Outport  Port=3
  wires:
  Sum4/1 -> Saturation1/1
  Saturation1/1 -> Vd/1
  I_d/1 -> Bus Creator/3, Sum2/2
  Sum3/1 -> Saturation3/1
  we/1 -> FFW/2(We)
  Gain1/1 -> PID_3/1(Fsw_out)
  I_d_ref/1 -> FFW/3(Id), Sum2/1  "Id_ref"
  FFW/1(Vq_FFW) -> Sum3/2
  Fsw_out/1 -> Gain1/1, Gain/1
  FFW/2(Vd_FFW) -> Sum4/1
  Bus Creator/1 -> Currents/1
  PID_3/1(v) -> Sum4/2
  PID_2/1(v) -> Sum3/1
  Gain/1 -> PID_2/2(Fsw_out)
  Sum1/1 -> PID_2/1(e)
  Saturation3/1 -> Vq/1
  Sum2/1 -> PID_3/2(e)
  Signal Builder1/1(Signal 1) -> Gain2/1  "Iq_ref"
  I_q/1 -> Bus Creator/1, Sum1/1
  Gain2/1 -> Bus Creator/2, FFW/1(Iq), Sum1/2

== system FieldControl_PID/Field_control_PID/Speed_control/Clark_Transformation1 ==
  Ia : Inport
  Ib : Inport  Port=2
  Ic : Inport  Port=3
  Add : Sum  Inputs=+++
  Add1 : Sum
  Gain : Gain  Gain=-0.5
  Gain1 : Gain  Gain=-0.5
  Gain2 : Gain  Gain=2/3
  Gain3 : Gain  Gain=sqrt(3)/2
  Gain4 : Gain  Gain=-sqrt(3)/2
  Gain5 : Gain  Gain=2/3
  I_alpha : Outport
  I_beta : Outport  Port=2
  wires:
  Gain5/1 -> I_beta/1
  Add1/1 -> Gain5/1
  Gain3/1 -> Add1/1
  Gain4/1 -> Add1/2
  Gain2/1 -> I_alpha/1
  Add/1 -> Gain2/1
  Ia/1 -> Add/1
  Gain1/1 -> Add/3
  Gain/1 -> Add/2
  Ic/1 -> Gain1/1, Gain4/1
  Ib/1 -> Gain/1, Gain3/1

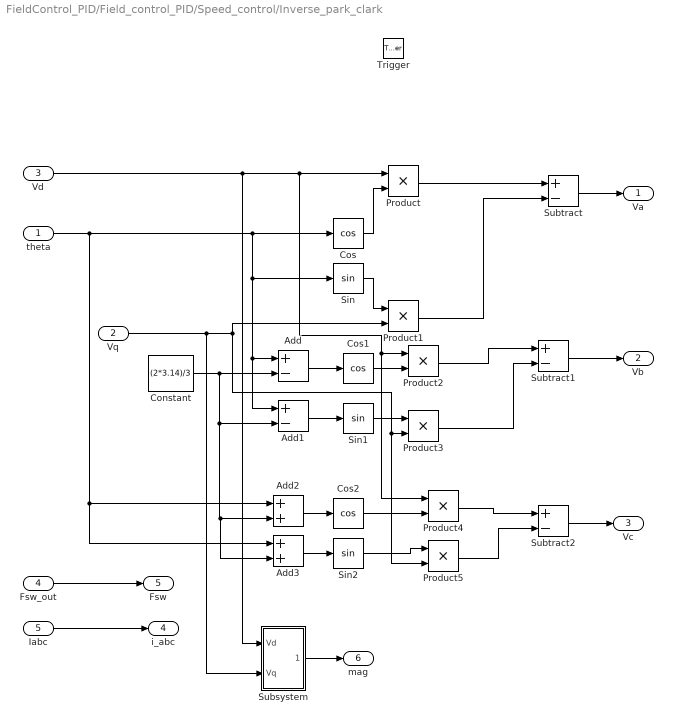
== system FieldControl_PID/Field_control_PID/Speed_control/Inverse_park_clark ==
  theta : Inport
  Vq : Inport  Port=2
  Vd : Inport  Port=3
  Fsw_out : Inport  Port=4
  Iabc : Inport  Port=5
  Trigger : TriggerPort  VariantControl=(inherit)
  Add : Sum  Inputs=+-
  Add1 : Sum  Inputs=+-
  Add2 : Sum
  Add3 : Sum
  Constant : Constant  Value=(2*3.14)/3
  Cos : Trigonometry  Operator=cos
  Cos1 : Trigonometry  Operator=cos
  Cos2 : Trigonometry  Operator=cos
  Product{,1..5} (6 alike) : Product
  Sin : Trigonometry
  Sin1 : Trigonometry
  Sin2 : Trigonometry
  Subsystem : Subsystem
  Subtract : Sum  Inputs=+-
  Subtract1 : Sum  Inputs=+-
  Subtract2 : Sum  Inputs=+-
  Va : Outport
  Vb : Outport  Port=2
  Vc : Outport  Port=3
  i_abc : Outport  Port=4
  Fsw : Outport  Port=5
  mag : Outport  Port=6
  wires:
  Add3/1 -> Sin2/1
  Add2/1 -> Cos2/1
  Sin2/1 -> Product5/1
  Cos2/1 -> Product4/2
  Product5/1 -> Subtract2/2
  Product4/1 -> Subtract2/1
  Subtract2/1 -> Vc/1
  Constant/1 -> Add/2, Add1/2, Add2/2, Add3/2
  Subtract1/1 -> Vb/1
  Product3/1 -> Subtract1/2
  Product2/1 -> Subtract1/1
  Sin1/1 -> Product3/1
  Cos1/1 -> Product2/2
  Add1/1 -> Sin1/1
  Add/1 -> Cos1/1
  Product1/1 -> Subtract/2
  Sin/1 -> Product1/1
  Vq/1 -> Subsystem/2(Vq), Product1/2, Product3/2, Product5/2
  Product/1 -> Subtract/1
  Cos/1 -> Product/2
  Vd/1 -> Subsystem/1(Vd), Product/1, Product2/1, Product4/1
  theta/1 -> Sin/1, Add/1, Add1/1, Cos/1, Add2/1, Add3/1
  Subtract/1 -> Va/1
  Iabc/1 -> i_abc/1
  Fsw_out/1 -> Fsw/1
  Subsystem/1(Out1) -> mag/1

== system FieldControl_PID/Field_control_PID/Speed_control/Inverter  ==
  "Switches " : Inport
  Fcn : Fcn  Expr=Vdc/3*(2*u(1)-u(2)-u(3))
  Fcn1 : Fcn  Expr=Vdc/3*(2*u(2)-u(1)-u(3))
  Fcn2 : Fcn  Expr=Vdc/3*(2*u(3)-u(2)-u(1))
  Mux1 : Mux  Inputs=3
  "Voltage " : Outport  VectorParamsAs1DForOutWhenUnconnected=off
  wires:
  Fcn2/1 -> Mux1/3
  Fcn/1 -> Mux1/1
  "Switches "/1 -> Fcn/1, Fcn1/1, Fcn2/1
  Fcn1/1 -> Mux1/2
  Mux1/1 -> "Voltage "/1

== system FieldControl_PID/Field_control_PID/Speed_control/PMSM ==
  Va : Inport
  Vb : Inport  Port=2
  Vc : Inport  Port=3
  Clark_Transformation : Subsystem
  Electrical_system2 : Subsystem
  Gain : Gain  Gain=P/2
  Integrator : Integrator
  Inverse_park_clark : Subsystem
  Mechanical_system : Subsystem
  Mux : Mux  Inputs=3
  Park_Transformation : Subsystem
      settings: PortSchema="{\"entries\":[{\"content\":{\"sides\":[{\"content\":{\"connectorIds\":[\"In1\",\"In2\"]},\"type\":\"ConnectorPlacement.EquallySpacedRectSide\",\"uuid\":\"a5303260-9056-4ba9-bf21-9d9e68c76aad\"},{\"content\":{\"connectorIds\":[\"Out1\",\"Out2\"],\"side\":\"RIGHT\"},\"type\":\"ConnectorPlacement.EquallySpacedRectSide\",\"uuid\":\"bf8eba39-f781-4672-b99d-9d1cb4b6396f\"},{\"content\":{\"connectorIds\":[],\"side\":\"TOP\"},\"type\":\"ConnectorPlacement.EquallySpacedRectSide\",\"uuid\":\"4985423e-053d-4914-82fe-b9dd9f427f0d\"},{\"content\":{\"connectorIds\":[\"In3\"],\"side\":\"BOTTOM\"},\"type\":\"ConnectorPlacement.EquallySpacedRectSide\",\"uuid\":\"0752c2be-c5bb-44b3-a6b0-4f5b66c2ccb1\"}]},\"type\":\"ConnectorPlacement.EquallySpacedConnector\",\"uuid\":\"0aeb7acd-9c9e-4bf3-9d65-4f157eb3bd0a\"}],\"packageUris\":[\"http://schema.mathworks.com/mf0/Connector/R2020b\"],\"version\":\"1.0\"}"
  Scope : Scope  NumInputPorts=2
  Scope1 : Scope  NumInputPorts=2
  Torque_system : Subsystem
  Stator_currents_Iabc : Outport
  Rotor_speed_Wm : Outport  Port=2
  Te : Outport  Port=3
  wires:
  Mux/1 -> Stator_currents_Iabc/1
  Inverse_park_clark/3(Ic) -> Mux/3  "Ic"
  Inverse_park_clark/2(Ib) -> Mux/2  "Ib"
  Inverse_park_clark/1(Ia) -> Mux/1  "Ia"
  Integrator/1 -> Park_Transformation/3(theta), Inverse_park_clark/1(theta)  "Rotor_angle_theta_elec"
  Gain/1 -> Integrator/1, Electrical_system2/3(W_e)  "We"
  Mechanical_system/1(Wm) -> Rotor_speed_Wm/1, Gain/1  "Wm"
  Torque_system/1(Te) -> Mechanical_system/1(Te), Te/1  "Te"
  Electrical_system2/2(I_q) -> Torque_system/2(I_q), Inverse_park_clark/2(Iq), Scope/1  "Iq"
  Electrical_system2/1(I_d) -> Inverse_park_clark/3(Id), Scope/2, Torque_system/1(I_d)  "Id"
  Park_Transformation/2(V_q) -> Scope1/2, Electrical_system2/2(V_q)  "Vq"
  Park_Transformation/1(V_d) -> Scope1/1, Electrical_system2/1(V_d)  "Vd"
  Clark_Transformation/2(V_beta) -> Park_Transformation/2(V_beta)
  Clark_Transformation/1(V_alpha) -> Park_Transformation/1(V_alpha)
  Vc/1 -> Clark_Transformation/3(Vc)
  Vb/1 -> Clark_Transformation/2(Vb)
  Va/1 -> Clark_Transformation/1(Va)

== system FieldControl_PID/Field_control_PID/Speed_control/Park_Transformation1 ==
  I_alpha : Inport
  I_beta : Inport  Port=2
  theta : Inport  Port=3
  Add : Sum
  Add1 : Sum
  Cos : Trigonometry  Operator=cos
  Cos1 : Trigonometry
  Gain : Gain  Gain=-1
  Product{,1..3} (4 alike) : Product
  I_d : Outport
  I_q : Outport  Port=2
  wires:
  Add1/1 -> I_q/1
  Product3/1 -> Add1/2
  Gain/1 -> Add1/1
  Product2/1 -> Gain/1
  Add/1 -> I_d/1
  Product1/1 -> Add/2
  Product/1 -> Add/1
  I_beta/1 -> Product1/2, Product3/1
  Cos1/1 -> Product1/1, Product2/2
  Cos/1 -> Product/2, Product3/2
  I_alpha/1 -> Product/1, Product2/1
  theta/1 -> Cos/1, Cos1/1

== system FieldControl_PID/Field_control_PID/Speed_control/SQ_Gen ==
  Clock : Clock
  Constant : Constant
  Divide : Product  Inputs=*/
  F : Constant  Value=500
  Gain1 : Gain  Gain=0.5
  Gain2 : Gain
  Mod : Math  Operator=mod  SaturateOnIntegerOverflow=on
  Relational Operator : RelationalOperator  Operator=<=  OutDataTypeStr=boolean  RndMeth=Simplest
  Cs : Outport
  wires:
  F/1 -> Gain2/1
  Clock/1 -> Mod/1
  Mod/1 -> Relational Operator/1
  Gain2/1 -> Divide/2
  Divide/1 -> Gain1/1, Mod/2
  Constant/1 -> Divide/1
  Gain1/1 -> Relational Operator/2
  Relational Operator/1 -> Cs/1

== system FieldControl_PID/Field_control_PID/Speed_control/SQ_gen ==
  F : Inport
  Clock : Clock
  Constant : Constant
  Divide : Product  Inputs=*/
  Gain1 : Gain  Gain=0.5
  Gain2 : Gain
  Mod : Math  Operator=mod  SaturateOnIntegerOverflow=on
  Relational Operator : RelationalOperator  Operator=<=  OutDataTypeStr=boolean  RndMeth=Simplest
  Cs : Outport
  wires:
  Relational Operator/1 -> Cs/1
  Gain1/1 -> Relational Operator/2
  Constant/1 -> Divide/1
  Divide/1 -> Mod/2, Gain1/1
  Gain2/1 -> Divide/2
  Mod/1 -> Relational Operator/1
  Clock/1 -> Mod/1
  F/1 -> Gain2/1

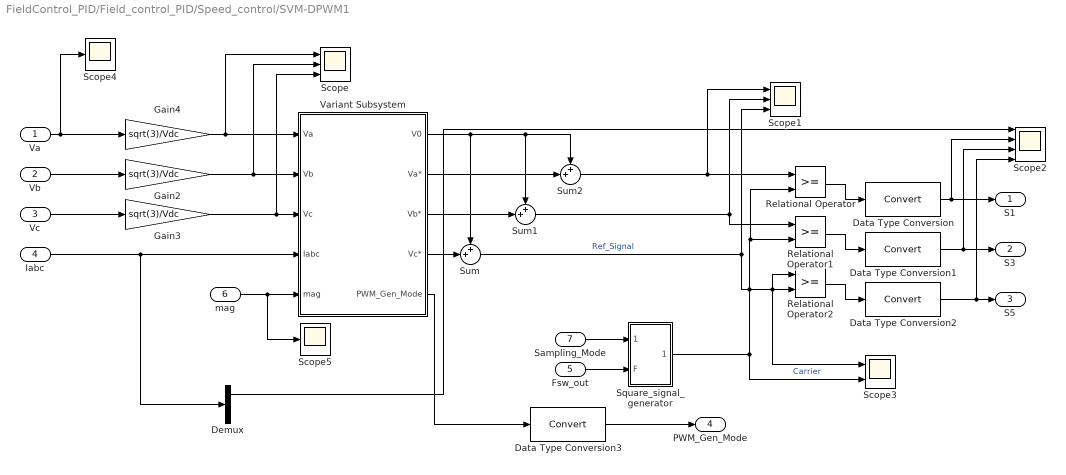
== system FieldControl_PID/Field_control_PID/Speed_control/SVM-DPWM1 ==
  Va : Inport
  Vb : Inport  Port=2
  Vc : Inport  Port=3
  Iabc : Inport  Port=4
  Fsw_out : Inport  Port=5
  mag : Inport  Port=6
  Sampling_Mode : Inport  Port=7
  Data Type Conversion{,1..3} (4 alike) : DataTypeConversion
  Demux : Demux  Outputs=3
  Gain2 : Gain  Gain=sqrt(3)/Vdc
  Gain3 : Gain  Gain=sqrt(3)/Vdc
  Gain4 : Gain  Gain=sqrt(3)/Vdc
  Relational Operator : RelationalOperator  OutDataTypeStr=boolean  RndMeth=Simplest
  Relational Operator1 : RelationalOperator  OutDataTypeStr=boolean  RndMeth=Simplest
  Relational Operator2 : RelationalOperator  OutDataTypeStr=boolean  RndMeth=Simplest
  Scope : Scope  NumInputPorts=3
  Scope1 : Scope  NumInputPorts=3
  Scope2 : Scope  NumInputPorts=4
  Scope3 : Scope  NumInputPorts=2
  Scope4 : Scope
  Scope5 : Scope
  Square_signal_generator : Subsystem
  Sum : Sum  Inputs=++|
  Sum1 : Sum  Inputs=++|
  Sum2 : Sum  Inputs=++|
  Variant Subsystem : Subsystem  Variant=on
  S1 : Outport
  S3 : Outport  Port=2
  S5 : Outport  Port=3
  PWM_Gen_Mode : Outport  Port=4  OutDataTypeStr=double
  wires:
  Data Type Conversion/1 -> Scope2/2, S1/1
  Data Type Conversion1/1 -> Scope2/3, S3/1
  Data Type Conversion2/1 -> Scope2/4, S5/1
  Relational Operator/1 -> Data Type Conversion/1
  Relational Operator1/1 -> Data Type Conversion1/1
  Relational Operator2/1 -> Data Type Conversion2/1
  Sum/1 -> Scope3/1, Relational Operator2/1, Scope1/3  "Ref_Signal"
  Sum1/1 -> Relational Operator1/1, Scope1/2
  Sum2/1 -> Relational Operator/1, Scope1/1
  Square_signal_generator/1(Output) -> Relational Operator/2, Relational Operator1/2, Relational Operator2/2, Scope3/2  "Carrier"
  Variant Subsystem/1(V0) -> Sum/1, Sum1/1, Sum2/1
  Va/1 -> Scope4/1, Gain4/1
  Vb/1 -> Gain2/1
  Vc/1 -> Gain3/1
  Variant Subsystem/2(Va*) -> Sum2/2
  Variant Subsystem/3(Vb*) -> Sum1/2
  Variant Subsystem/4(Vc*) -> Sum/2
  Sampling_Mode/1 -> Square_signal_generator/1(Mode)
  Fsw_out/1 -> Square_signal_generator/2(F)
  Iabc/1 -> Demux/1, Variant Subsystem/4(Iabc)
  Gain4/1 -> Scope/1, Variant Subsystem/1(Va)
  Gain2/1 -> Scope/2, Variant Subsystem/2(Vb)
  Gain3/1 -> Scope/3, Variant Subsystem/3(Vc)
  Demux/1 -> Scope2/1
  mag/1 -> Scope5/1, Variant Subsystem/5(mag)
  Variant Subsystem/5(PWM_Gen_Mode) -> Data Type Conversion3/1
  Data Type Conversion3/1 -> PWM_Gen_Mode/1

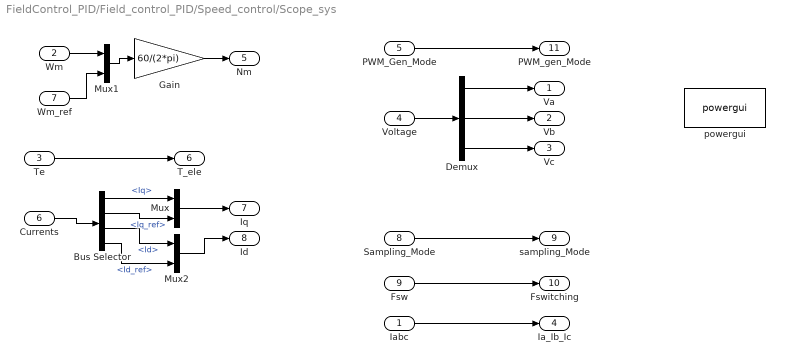
== system FieldControl_PID/Field_control_PID/Speed_control/Scope_sys ==
  Iabc : Inport
  Wm : Inport  Port=2
  Te : Inport  Port=3
  "Voltage " : Inport  Port=4
  PWM_Gen_Mode : Inport  Port=5
  Currents : Inport  Port=6
  Wm_ref : Inport  Port=7
  Sampling_Mode : Inport  Port=8
  Fsw : Inport  Port=9
  Bus Selector : BusSelector  OutputSignals=Iq,Iq_ref,Id,Id_ref
  Demux : Demux  Outputs=3
  Gain : Gain  Gain=60/(2*pi)
  Mux : Mux  Inputs=2
  Mux1 : Mux  Inputs=2
  Mux2 : Mux  Inputs=2
  powergui : spspowerguiLib/powergui  Priority=1  SimulationMode=Continuous  SampleTime=50e-6  frequency=60  Iterations=50  frequencyindice=60  Pbase=100e6  ErrMax=1e-4  UnitsV=kV  UnitsW=MW  buscounter=0  FunctionMessages=off  echomessages=off  EnableUseOfTLC=off  CurrentSourceSwitches=off  DisableSnubberDevices=off  DisableRonSwitches=off  DisableVfSwitches=off  DisplayEquations=off  AutomaticDiscreteSolvers=off  SolverType=Tustin/Backward Euler (TBE)  Interpol=off  ExternalGateDelay=off  methode=off  Ts=100  x0status=blocks  SPID=on  SwTol=0  HookPort=off  NonlinearTolerance=1e-4  nMaxIteration=100  ContinueOnMaxIteration=off  RestoreLinks=warning  ResistiveCurrentMeasurement=off  Frange=[0:2:500]  Ylog=off  Xlog=on  ShowGrid=off  save=off  variable=ZData  structure=0  ZoomFFT=off  StartTime=0.0  cycles=1  DisplayStyle=1  fundamental=60  FreqAxis=off  MaxFrequency=1000  frequencyindicesteady=1  RmsSteady=1  display=off
  Va : Outport
  Vb : Outport  Port=2
  Vc : Outport  Port=3
  Ia_Ib_Ic : Outport  Port=4
  Nm : Outport  Port=5
  T_ele : Outport  Port=6
  Iq : Outport  Port=7
  "Id " : Outport  Port=8
  sampling_Mode : Outport  Port=9
  Fswitching : Outport  Port=10
  PWM_gen_Mode : Outport  Port=11
  wires:
  Mux/1 -> Iq/1
  Bus Selector/2 -> Mux/2  "<Iq_ref>"
  Bus Selector/1 -> Mux/1  "<Iq>"
  Currents/1 -> Bus Selector/1
  Te/1 -> T_ele/1
  Gain/1 -> Nm/1
  Iabc/1 -> Ia_Ib_Ic/1
  Demux/3 -> Vc/1
  Demux/2 -> Vb/1
  Demux/1 -> Va/1
  "Voltage "/1 -> Demux/1
  Fsw/1 -> Fswitching/1
  Sampling_Mode/1 -> sampling_Mode/1
  Mux1/1 -> Gain/1
  Wm/1 -> Mux1/1
  Wm_ref/1 -> Mux1/2
  Bus Selector/3 -> Mux2/1  "<Id>"
  Bus Selector/4 -> Mux2/2  "<Id_ref>"
  Mux2/1 -> "Id "/1
  PWM_Gen_Mode/1 -> PWM_gen_Mode/1

== system FieldControl_PID/Field_control_PID/Speed_control/Triggered Speed_Control ==
  Wm : Inport
  Trigger : TriggerPort  VariantControl=(inherit)
  Constant : Constant  Value=500
  Gain1 : Gain  Gain=350
  MTPA : Subsystem  Variant=on
  PI_system3 : Subsystem
  Signal Builder2 : Subsystem  Tag=STV Subsys  LoadFcn=sigbuilder_block('load');  StartFcn=sigbuilder_block('start');  StopFcn=sigbuilder_block('stop');  ClipboardFcn=sigbuilder_block('clipboard');  mask(Sigbuilder block){tuvar=[0:10]}
      mask help: Simulink:masks:SigbuilderBlock_MD
      mask init:
      | if ~strcmp(get_param(bdroot(gcbh),'SimulationStatus'),'stopped') tuvar = sigbuilder_block('maskInit'); end
      settings: CopyFcn=sigbuilder_block('copy');  DeleteFcn=sigbuilder_block('delete');  ModelCloseFcn=sigbuilder_block('modelClose');  PreSaveFcn=sigbuilder_block('preSave');  PauseFcn=sigbuilder_block('pause');  ContinueFcn=sigbuilder_block('continue');  NameChangeFcn=sigbuilder_block('namechange');  OpenFcn=sigbuilder_block('open',[5.4 30 1141.2 522.6 ]);  CloseFcn=sigbuilder_block('close');
      mask Display: plot(0, 0, 100, 100,[2, 2, 32, 32, 2], [68, 8, 8, 68, 68],[32, 2], [38, 38], [32, 19, 2],[53, 60, 44], [32, 17, 17, 2],[16, 16, 31, 31]);txt = getActiveGroup(gcbh);text(2, 100, txt,'verticalAlignment', 'top');
  Some_Edits : Subsystem  Commented=on
  Sum : Sum  Inputs=|+-
  Switching_Frequency : Subsystem
  SM : Outport
  Fsw : Outport  Port=2
  Id_ref : Outport  Port=3
  Iq_ref : Outport  Port=4
  Wm_ref : Outport  Port=5
  wires:
  MTPA/1(Id_ref) -> Id_ref/1
  MTPA/2(Iq_ref) -> Iq_ref/1
  Wm/1 -> Sum/2
  PI_system3/1(T_ref) -> MTPA/1(Tref)
  Gain1/1 -> Switching_Frequency/1(Wm), Sum/1, Wm_ref/1
  Sum/1 -> PI_system3/1(Error)
  Signal Builder2/1(Signal 1) -> Gain1/1  "Wm"
  Switching_Frequency/1(Fsw_out) -> Fsw/1
  Switching_Frequency/2(Sampling_Mode) -> SM/1

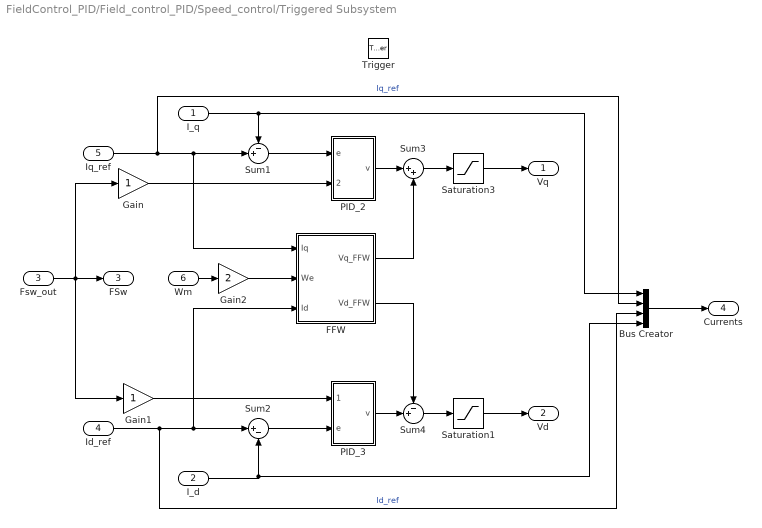
== system FieldControl_PID/Field_control_PID/Speed_control/Triggered Subsystem ==
  I_q : Inport
  I_d : Inport  Port=2
  Fsw_out : Inport  Port=3
  Id_ref : Inport  Port=4
  Iq_ref : Inport  Port=5
  Wm : Inport  Port=6
  Trigger : TriggerPort  VariantControl=(inherit)
  Bus Creator : BusCreator  Inputs=4
  FFW : Subsystem
  Gain : Gain
  Gain1 : Gain
  Gain2 : Gain  Gain=2
  PID_2 : Subsystem
  PID_3 : Subsystem
  Saturation1 : Saturate  UpperLimit=Vdc/sqrt(3)  LowerLimit=-Vdc/sqrt(3)
  Saturation3 : Saturate  UpperLimit=Vdc/sqrt(3)  LowerLimit=-Vdc/sqrt(3)
  Sum1 : Sum  Inputs=-+|
  Sum2 : Sum  Inputs=|+-
  Sum3 : Sum  Inputs=|++
  Sum4 : Sum  Inputs=-+|
  Vq : Outport
  Vd : Outport  Port=2
  FSw : Outport  Port=3
  Currents : Outport  Port=4
  wires:
  Bus Creator/1 -> Currents/1
  Iq_ref/1 -> Bus Creator/2, FFW/1(Iq), Sum1/2  "Iq_ref"
  I_q/1 -> Bus Creator/1, Sum1/1
  Sum1/1 -> PID_2/1(e)
  PID_2/1(v) -> Sum3/1
  Sum3/1 -> Saturation3/1
  Saturation3/1 -> Vq/1
  I_d/1 -> Bus Creator/4, Sum2/2
  Id_ref/1 -> Bus Creator/3, FFW/3(Id), Sum2/1  "Id_ref"
  Saturation1/1 -> Vd/1
  Sum4/1 -> Saturation1/1
  PID_3/1(v) -> Sum4/2
  Sum2/1 -> PID_3/2(e)
  Gain2/1 -> FFW/2(We)
  FFW/2(Vd_FFW) -> Sum4/1
  FFW/1(Vq_FFW) -> Sum3/2
  Fsw_out/1 -> Gain1/1, Gain/1, FSw/1
  Gain/1 -> PID_2/2(Fsw_out)
  Gain1/1 -> PID_3/1(Fsw_out)
  Wm/1 -> Gain2/1

== system FieldControl_PID/Field_control_PID/Current_control/Inverse_park_clark/Subsystem ==
  Vd : Inport
  Vq : Inport  Port=2
  Add : Sum
  Square : Math  Operator=square  SaturateOnIntegerOverflow=on
  Square Root : Sqrt  SaturateOnIntegerOverflow=on
  Square1 : Math  Operator=square  SaturateOnIntegerOverflow=on
  mag : Outport
  wires:
  Square1/1 -> Add/1
  Add/1 -> Square Root/1
  Vd/1 -> Square1/1
  Square/1 -> Add/2
  Square Root/1 -> mag/1
  Vq/1 -> Square/1
